simulink subsystem "CONTROL_DESATURATION"  (R2025b)
settings: Solver=VariableStepAuto  StartTime=0.0  StopTime=10.0  RelTol=1e-3
undefined symbols (not defined in the file): desatK, mtqAllocationMatrix, mtqMagneticGain, mtqMaxMagDip, mtqResistance, rwInertia
libraries: matrix_library x2, vrlib x1
settings Model: Creator=antoniohernandez-rodiciomateos  LastModifiedBy=antoniohernandez-rodiciomateos

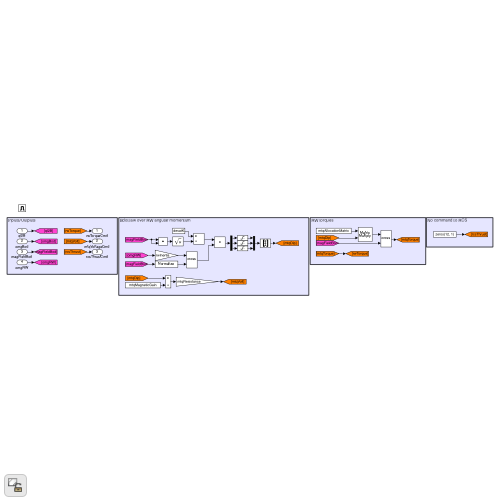
[thumbnail: Simulink's stored preview of the top-level diagram]
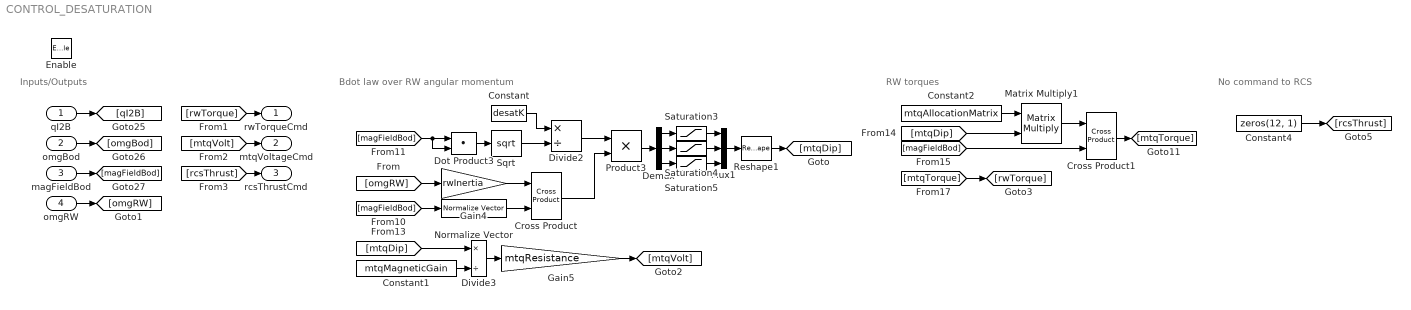
== system CONTROL_DESATURATION ==
  note: Inputs/Outputs
  note: No command to RCS
  note: Bdot law over RW angular momentum
  note: RW torques
  qI2B : Inport  OutDataTypeStr=double  PortDimensions=[4 1]
  omgBod : Inport  Port=2  OutDataTypeStr=double  PortDimensions=[3 1]
  magFieldBod : Inport  Port=3  OutDataTypeStr=double  PortDimensions=[3 1]
  omgRW : Inport  Port=4  OutDataTypeStr=double  PortDimensions=[3 1]
  Enable : EnablePort
  Constant : Constant  Value=desatK
  Constant1 : Constant  Value=mtqMagneticGain
  Constant2 : Constant  Value=mtqAllocationMatrix
  Constant4 : Constant  Value=zeros(12, 1)
  Cross Product : matrix_library/Cross Product
  Cross Product1 : matrix_library/Cross Product
  Demux : Demux  Outputs=3
  Divide2 : Product  Inputs=*/
  Divide3 : Product  Inputs=*/
  Dot Product3 : DotProduct  OutDataTypeStr=Inherit: Inherit via internal rule
  Gain4 : Gain  Gain=rwInertia
  Gain5 : Gain  Gain=mtqResistance
  Matrix Multiply1 : Product  Multiplication=Matrix(*)
  Mux1 : Mux  Inputs=3
  Normalize Vector : vrlib/Utilities/Normalize Vector  maxzero=0
  Product3 : Product
  Reshape1 : Reshape  OutputDimensionality=Column vector (2-D)
  Saturation3 : Saturate  UpperLimit=mtqMaxMagDip(1)  LowerLimit=-1 * mtqMaxMagDip(1)
  Saturation4 : Saturate  UpperLimit=mtqMaxMagDip(2)  LowerLimit=-1 * mtqMaxMagDip(2)
  Saturation5 : Saturate  UpperLimit=mtqMaxMagDip(3)  LowerLimit=-1 * mtqMaxMagDip(3)
  Sqrt : Sqrt
  rwTorqueCmd : Outport  OutDataTypeStr=double  PortDimensions=[3 1]
  mtqVoltageCmd : Outport  Port=2  OutDataTypeStr=double  PortDimensions=[3 1]
  rcsThrustCmd : Outport  Port=3  OutDataTypeStr=double  PortDimensions=[12 1]
  wires:
  [rcsThrust] -> rcsThrustCmd/1
  [mtqVolt] -> mtqVoltageCmd/1
  [rwTorque] -> rwTorqueCmd/1
  omgBod/1 -> [omgBod]
  magFieldBod/1 -> [magFieldBod]
  qI2B/1 -> [qI2B]
  omgRW/1 -> [omgRW]
  Sqrt/1 -> Divide2/2
  Normalize Vector/1 -> Cross Product/2
  Reshape1/1 -> [mtqDip]
  Demux/3 -> Saturation5/1
  Gain4/1 -> Cross Product/1
  Demux/1 -> Saturation3/1
  Dot Product3/1 -> Sqrt/1
  Saturation3/1 -> Mux1/1
  Saturation5/1 -> Mux1/3
  [magFieldBod] -> Normalize Vector/1
  Cross Product/1 -> Product3/2
  Saturation4/1 -> Mux1/2
  Divide2/1 -> Product3/1
  Product3/1 -> Demux/1
  [omgRW] -> Gain4/1
  Demux/2 -> Saturation4/1
  Mux1/1 -> Reshape1/1
  [magFieldBod] -> Dot Product3/2, Dot Product3/1
  Constant/1 -> Divide2/1
  Constant1/1 -> Divide3/2
  Divide3/1 -> Gain5/1
  [mtqDip] -> Divide3/1
  Gain5/1 -> [mtqVolt]
  [mtqDip] -> Matrix Multiply1/2
  [magFieldBod] -> Cross Product1/2
  Matrix Multiply1/1 -> Cross Product1/1
  Constant2/1 -> Matrix Multiply1/1
  Cross Product1/1 -> [mtqTorque]
  [mtqTorque] -> [rwTorque]
  Constant4/1 -> [rcsThrust]
